simulink model "staticNoiseSimulation"  (R2016b)
settings: Solver=FixedStepAuto  StartTime=0.0  StopTime=T  FixedStep=Ta  RelTol=1e-3
InitFcn:
  | initSim
StopFcn:
  | endSim
undefined symbols (not defined in the file): n_power, phi
libraries: simulink x1
settings Model: Creator=ich  LastModifiedBy=ich

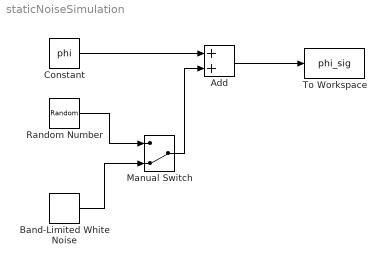
== system staticNoiseSimulation ==
  Add : Sum
  Band-Limited White Noise : simulink/Sources/Band-Limited White Noise  Cov=[n_power]  Ts=0.02  seed=[23341]
  Constant : Constant  Value=phi
  Manual Switch : ManualSwitch  CurrentSetting=0
  Random Number : RandomNumber  Variance=23  SampleTime=0.02
  To Workspace : ToWorkspace  VariableName=phi_sig  SaveFormat=Timeseries  SampleTime=-1
  wires:
  Constant/1 -> Add/1
  Add/1 -> To Workspace/1
  Random Number/1 -> Manual Switch/1
  Band-Limited White Noise/1 -> Manual Switch/2
  Manual Switch/1 -> Add/2
